simulink model "mpm_blocks"  (R2023a)
settings: Solver=VariableStepAuto  StartTime=0.0  StopTime=10.0  RelTol=1e-3
undefined symbols (not defined in the file or in its folder): conv, es
(part 3 of 3)

== system mpm_blocks/MOSFET w// Integrated Diode 2-Level VSC/Thermal Model/Subsystem4 ==
  P : Inport
  THS : Inport  Port=2
  Gain : Gain  Gain=1/(conv.dev(1).theta(4)+conv.theta(1))
  Gain1 : Gain  Gain=1/conv.dev(1).theta(3)
  Gain11 : Gain  Gain=1/conv.dev(1).c(1)
  Gain2 : Gain  Gain=1/conv.dev(1).c(4)
  Gain3 : Gain  Gain=1/conv.dev(1).theta(3)
  Gain4 : Gain  Gain=1/conv.dev(1).theta(2)
  Gain5 : Gain  Gain=1/conv.dev(1).c(3)
  Gain6 : Gain  Gain=1/conv.dev(1).theta(2)
  Gain7 : Gain  Gain=1/conv.dev(1).theta(1)
  Gain8 : Gain  Gain=1/conv.dev(1).c(2)
  Gain9 : Gain  Gain=1/conv.dev(1).theta(1)
  Integrator{,1..3} (4 alike) : Integrator  InitialCondition=conv.T_init-273.15
  Subtract{,1..9,11} (11 alike) : Sum  Inputs=+-
  T_c : Outport
  T_j : Outport  Port=2
  wires:
  [T2] -> Subtract4/1, Subtract6/1, Subtract7/2, Subtract9/2  "T2"
  Gain/1 -> Subtract2/2
  Subtract5/1 -> Gain5/1
  Gain4/1 -> Subtract5/1
  Subtract3/1 -> Gain3/1
  Gain8/1 -> Integrator1/1  "d_T2"
  Integrator/1 -> T_j/1, [T1]  "T1"
  [T3] -> Subtract1/1, Subtract3/1, Subtract4/2, Subtract6/2  "T3"
  P/1 -> Subtract11/1
  Subtract9/1 -> Gain9/1
  Subtract1/1 -> Gain1/1
  [T1] -> Subtract9/1, Subtract7/1  "T1"
  Integrator1/1 -> [T2]  "T2"
  Subtract/1 -> Gain/1
  [T4] -> Subtract/1, Subtract1/2, Subtract3/2  "T4"
  Subtract7/1 -> Gain7/1
  Subtract4/1 -> Gain4/1
  Integrator3/1 -> [T4], T_c/1  "T4"
  Gain2/1 -> Integrator3/1  "d_T4"
  Subtract8/1 -> Gain8/1
  THS/1 -> Subtract/2
  Gain1/1 -> Subtract2/1
  Gain9/1 -> Subtract11/2
  Gain3/1 -> Subtract5/2
  Integrator2/1 -> [T3]  "T3"
  Gain5/1 -> Integrator2/1  "d_T3"
  Gain11/1 -> Integrator/1  "d_T1"
  Subtract2/1 -> Gain2/1
  Subtract6/1 -> Gain6/1
  Subtract11/1 -> Gain11/1
  Gain7/1 -> Subtract8/1
  Gain6/1 -> Subtract8/2

== system mpm_blocks/MOSFET w// Integrated Diode 2-Level VSC/Thermal Model/Subsystem5 ==
  P : Inport
  THS : Inport  Port=2
  Gain : Gain  Gain=1/(conv.dev(1).theta(4)+conv.theta(1))
  Gain1 : Gain  Gain=1/conv.dev(1).theta(3)
  Gain11 : Gain  Gain=1/conv.dev(1).c(1)
  Gain2 : Gain  Gain=1/conv.dev(1).c(4)
  Gain3 : Gain  Gain=1/conv.dev(1).theta(3)
  Gain4 : Gain  Gain=1/conv.dev(1).theta(2)
  Gain5 : Gain  Gain=1/conv.dev(1).c(3)
  Gain6 : Gain  Gain=1/conv.dev(1).theta(2)
  Gain7 : Gain  Gain=1/conv.dev(1).theta(1)
  Gain8 : Gain  Gain=1/conv.dev(1).c(2)
  Gain9 : Gain  Gain=1/conv.dev(1).theta(1)
  Integrator{,1..3} (4 alike) : Integrator  InitialCondition=conv.T_init-273.15
  Subtract{,1..9,11} (11 alike) : Sum  Inputs=+-
  T_c : Outport
  T_j : Outport  Port=2
  wires:
  [T2] -> Subtract4/1, Subtract6/1, Subtract7/2, Subtract9/2  "T2"
  Gain/1 -> Subtract2/2
  Subtract5/1 -> Gain5/1
  Gain4/1 -> Subtract5/1
  Subtract3/1 -> Gain3/1
  Gain8/1 -> Integrator1/1  "d_T2"
  Integrator/1 -> T_j/1, [T1]  "T1"
  [T3] -> Subtract1/1, Subtract3/1, Subtract4/2, Subtract6/2  "T3"
  P/1 -> Subtract11/1
  Subtract9/1 -> Gain9/1
  Subtract1/1 -> Gain1/1
  [T1] -> Subtract9/1, Subtract7/1  "T1"
  Integrator1/1 -> [T2]  "T2"
  Subtract/1 -> Gain/1
  [T4] -> Subtract/1, Subtract1/2, Subtract3/2  "T4"
  Subtract7/1 -> Gain7/1
  Subtract4/1 -> Gain4/1
  Integrator3/1 -> [T4], T_c/1  "T4"
  Gain2/1 -> Integrator3/1  "d_T4"
  Subtract8/1 -> Gain8/1
  THS/1 -> Subtract/2
  Gain1/1 -> Subtract2/1
  Gain9/1 -> Subtract11/2
  Gain3/1 -> Subtract5/2
  Integrator2/1 -> [T3]  "T3"
  Gain5/1 -> Integrator2/1  "d_T3"
  Gain11/1 -> Integrator/1  "d_T1"
  Subtract2/1 -> Gain2/1
  Subtract6/1 -> Gain6/1
  Subtract11/1 -> Gain11/1
  Gain7/1 -> Subtract8/1
  Gain6/1 -> Subtract8/2

== system mpm_blocks/MOSFET w// Integrated Diode 2-Level VSC/Thermal Model/Subsystem6 ==
  P : Inport
  THS : Inport  Port=2
  Gain : Gain  Gain=1/(conv.dev(1).theta(4)+conv.theta(1))
  Gain1 : Gain  Gain=1/conv.dev(1).theta(3)
  Gain11 : Gain  Gain=1/conv.dev(1).c(1)
  Gain2 : Gain  Gain=1/conv.dev(1).c(4)
  Gain3 : Gain  Gain=1/conv.dev(1).theta(3)
  Gain4 : Gain  Gain=1/conv.dev(1).theta(2)
  Gain5 : Gain  Gain=1/conv.dev(1).c(3)
  Gain6 : Gain  Gain=1/conv.dev(1).theta(2)
  Gain7 : Gain  Gain=1/conv.dev(1).theta(1)
  Gain8 : Gain  Gain=1/conv.dev(1).c(2)
  Gain9 : Gain  Gain=1/conv.dev(1).theta(1)
  Integrator{,1..3} (4 alike) : Integrator  InitialCondition=conv.T_init-273.15
  Subtract{,1..9,11} (11 alike) : Sum  Inputs=+-
  T_c : Outport
  T_j : Outport  Port=2
  wires:
  [T2] -> Subtract4/1, Subtract6/1, Subtract7/2, Subtract9/2  "T2"
  Gain/1 -> Subtract2/2
  Subtract5/1 -> Gain5/1
  Gain4/1 -> Subtract5/1
  Subtract3/1 -> Gain3/1
  Gain8/1 -> Integrator1/1  "d_T2"
  Integrator/1 -> T_j/1, [T1]  "T1"
  [T3] -> Subtract1/1, Subtract3/1, Subtract4/2, Subtract6/2  "T3"
  P/1 -> Subtract11/1
  Subtract9/1 -> Gain9/1
  Subtract1/1 -> Gain1/1
  [T1] -> Subtract9/1, Subtract7/1  "T1"
  Integrator1/1 -> [T2]  "T2"
  Subtract/1 -> Gain/1
  [T4] -> Subtract/1, Subtract1/2, Subtract3/2  "T4"
  Subtract7/1 -> Gain7/1
  Subtract4/1 -> Gain4/1
  Integrator3/1 -> [T4], T_c/1  "T4"
  Gain2/1 -> Integrator3/1  "d_T4"
  Subtract8/1 -> Gain8/1
  THS/1 -> Subtract/2
  Gain1/1 -> Subtract2/1
  Gain9/1 -> Subtract11/2
  Gain3/1 -> Subtract5/2
  Integrator2/1 -> [T3]  "T3"
  Gain5/1 -> Integrator2/1  "d_T3"
  Gain11/1 -> Integrator/1  "d_T1"
  Subtract2/1 -> Gain2/1
  Subtract6/1 -> Gain6/1
  Subtract11/1 -> Gain11/1
  Gain7/1 -> Subtract8/1
  Gain6/1 -> Subtract8/2

== matlab function mpm_blocks/MOSFET w// Integrated Diode 2-Level VSC/Calculate Duty & Currents/Duty Cycle Estimation/MATLAB Function3 ==
  data: u input; y output
function y = checkMa(u)

if u > 1
    error('Modulation index (ma) greater than 1.');
end

y = u;

== matlab function mpm_blocks/MOSFET w// External Diode 2-Level VSC/Calculate Duty & Currents/Calculate Device Currents ==
  data: d_M input; d_deadTime input; i_s input; r_ds input; v_th input; r_dio input; i_M output size=[6 1]; i_D output size=[6 1]; d_D output
function [i_M, i_D, d_D]  = calcDevCurrent(d_M, d_deadTime, i_s, r_ds, v_th, r_dio)
%% Housekeeping
i_M = zeros(6,1);
i_D = zeros(6,1); 
d_D = zeros(6,1);
est_error = zeros(6,1);

v_ds_H = i_s .* r_ds(1:3); 
v_ds_L = -i_s .* r_ds(4:6); 

v_ds = [v_ds_H; v_ds_L];

%% A-Phase Devices 
% Devices (1) and (4)
% High-side
if(-v_ds(1) < v_th(1))
    i_M(1) = i_s(1); 
    i_D(1) = 0; 
    d_D(1) = d_deadTime;
else
    i_D(1) = -(i_s(1)*r_ds(1) + v_th(1)) / (r_ds(1) + r_dio(1));
    i_M(1) = i_s(1) + i_D(1); 
    d_D(1) = d_deadTime + d_M(1);
end

% Low-side
if(-v_ds(4) < v_th(4))
    i_M(4) = -i_s(1); 
    i_D(4) = 0; 
    d_D(4) = d_deadTime;
else
    i_D(4) = -(-i_s(1)*r_ds(4) + v_th(4)) / (r_ds(4) + r_dio(4));
    i_M(4) = i_D(4) - i_s(1); 
    d_D(4) = d_deadTime + d_M(4);
end

%% B-Phase Devices
% Devices (2) and (5)
% High-side
if(-v_ds(2) < v_th(2))
    i_M(2) = i_s(2); 
    i_D(2) = 0; 
    d_D(2) = d_deadTime;
else
    i_D(2) = -(i_s(2)*r_ds(2) + v_th(2)) / (r_ds(2) + r_dio(2));
    i_M(2) = i_s(2) + i_D(2); 
    d_D(2) = d_deadTime + d_M(2); 
end

% Low-side
if(-v_ds(5) < v_th(5))
    i_M(5) = -i_s(2); 
    i_D(5) = 0; 
    d_D(5) = d_deadTime; 
else
    i_D(5) = -(-i_s(2)*r_ds(5) + v_th(5)) / (r_ds(5) + r_dio(5));
    i_M(5) = i_D(5) - i_s(2); 
    d_D(5) = d_deadTime + d_M(5);
end

%% C-Phase Devices
% Devices (3) and (6)
% High-side
if(-v_ds(3) < v_th(3))
    i_M(3) = i_s(3); 
    i_D(3) = 0; 
    d_D(3) = d_deadTime; 
else
    i_D(3) = -(i_s(3)*r_ds(3) + v_th(3)) / (r_ds(3) + r_dio(3));
    i_M(3) = i_s(3) + i_D(3); 
    d_D(3) = d_deadTime + d_M(3); 
end

% Low-side
if(-v_ds(6) < v_th(3))
    i_M(6) = -i_s(3); 
    i_D(6) = 0; 
    d_D(6) = d_deadTime; 
else
    i_D(6) = -(-i_s(3)*r_ds(6) + v_th(6)) / (r_ds(6) + r_dio(6));
    i_M(6) = i_D(6) - i_s(3); 
    d_D(6) = d_deadTime + d_M(6); 
end

%% Calculate Error
for i = 1:3
    est_error(i) = i_s(i) - (i_M(i) - i_D(i));
    est_error(i+3) = i_s(i) + (i_M(i+3) - i_D(i+3));

    if(abs(est_error(i)/i_s(i)) > 0.2)
        error("CURRENT ESTIMATION ERROR: Estimation error for Device %d is greater than 20 percent", i)
    elseif(abs(est_error(i+3)/i_s(i)) > 0.2)
        error("CURRENT ESTIMATION ERROR: Estimation error for Device %d is greater than 20 percent", i)
    end
end

end

== matlab function mpm_blocks/IGBT 2-Level VSC2/Duty & Current Calculation/Calculate Device Currents ==
  data: d_Q input; d_deadTime input; i_s input; i_Q output size=[6 1]; d_Qnew output; i_D output size=[6 1]; d_D output
function [i_Q, d_Qnew, i_D, d_D]  = calcDevCurrent(d_Q, d_deadTime, i_s)
%% Housekeeping
i_Q = zeros(6,1);
i_D = zeros(6,1); 
d_D = zeros(6,1);
d_Qnew = zeros(6,1); 

% Calculating Device Currents
for i = 1:3
    if(i_s(i) > 0)
        % High-side device currents
        i_Q(i) = i_s(i); 
        i_D(i) = 0; 

        % Low-side device currents
        i_Q(i+3) = 0; 
        i_D(i+3) = i_s(i);

        % Diode duty cycle estimate
        d_Qnew(i) = d_Q(i);
        d_D(i) = 0;
        d_Qnew(i+3) = 0; 
        d_D(i+3) = d_Q(i+3) + d_deadTime;
    else
        % High-side device currents
        i_Q(i) = 0; 
        i_D(i) = -i_s(i); 

        % Low-side device currents
        i_Q(i+3) = -i_s(i); 
        i_D(i+3) = 0;

        % Diode duty cycle estimate
        d_Qnew(i) = 0; 
        d_D(i) = d_Q(i) + d_deadTime;
        d_Qnew(i+3) = d_Q(i+3);
        d_D(i+3) = 0; 
    end
end

== matlab function mpm_blocks/IGBT 2-Level VSC2/Duty & Current Calculation/MATLAB Function3 ==
  data: u input; y output
function y = checkMa(u)

if u > 1
    error('Modulation index (ma) greater than 1.');
end

y = u;

== matlab function mpm_blocks/MOSFET w// External Diode 2-Level VSC/Calculate Duty & Currents/Duty Cycle Estimation/MATLAB Function ==
  data: d1 input; d2 input; d3 input
function dutyCheck(d1, d2, d3)

if (d1+d2+d3 ~= 1)
    error("DUTY RATIO ERROR: check duty cycle function block")
end

== matlab function mpm_blocks/MOSFET w// External Diode 2-Level VSC/Calculate Duty & Currents/Duty Cycle Estimation/MATLAB Function3 ==
  data: u input; y output
function y = checkMa(u)

if u > 1
    error('Modulation index (ma) greater than 1.');
end

y = u;

== matlab function mpm_blocks/MOSFET w// Integrated Diode 2-Level VSC/Calculate Duty & Currents/Calculate Device Currents ==
  data: d_m input; d_d input; i_s input; r_ds input; v_th input; r_dio input; i_m output size=[6 1]; i_d output size=[6 1]; d_d_new output
function [i_m, i_d, d_d_new]  = calcDevCurrent(d_m, d_d, i_s, r_ds, v_th, r_dio)
%% Housekeeping
i_m = zeros(6,1);
i_d = zeros(6,1); 
d_d_new = zeros(6,1);
est_error = zeros(6,1);

v_ds_H = i_s .* r_ds(1:3); 
v_ds_L = -i_s .* r_ds(4:6); 

v_ds = [v_ds_H; v_ds_L];

%% A-Phase Devices 
% Devices (1) and (4)
% High-side
if(-v_ds(1) < v_th(1))
    i_m(1) = i_s(1); 
    i_d(1) = 0; 
    d_d_new(1) = d_d;
else
    i_d(1) = -(i_s(1)*r_ds(1) + v_th(1)) / (r_ds(1) + r_dio(1));
    i_m(1) = i_s(1) + i_d(1); 
    d_d_new(1) = d_d + d_m(1);
end

% Low-side
if(-v_ds(4) < v_th(4))
    i_m(4) = -i_s(1); 
    i_d(4) = 0; 
    d_d_new(4) = d_d;
else
    i_d(4) = -(-i_s(1)*r_ds(4) + v_th(4)) / (r_ds(4) + r_dio(4));
    i_m(4) = i_d(4) - i_s(1); 
    d_d_new(4) = d_d + d_m(4);
end

%% B-Phase Devices
% Devices (2) and (5)
% High-side
if(-v_ds(2) < v_th(2))
    i_m(2) = i_s(2); 
    i_d(2) = 0; 
    d_d_new(2) = d_d;
else
    i_d(2) = -(i_s(2)*r_ds(2) + v_th(2)) / (r_ds(2) + r_dio(2));
    i_m(2) = i_s(2) + i_d(2); 
    d_d_new(2) = d_d + d_m(2); 
end

% Low-side
if(-v_ds(5) < v_th(5))
    i_m(5) = -i_s(2); 
    i_d(5) = 0; 
    d_d_new(5) = d_d; 
else
    i_d(5) = -(-i_s(2)*r_ds(5) + v_th(5)) / (r_ds(5) + r_dio(5));
    i_m(5) = i_d(5) - i_s(2); 
    d_d_new(5) = d_d + d_m(5);
end

%% C-Phase Devices
% Devices (3) and (6)
% High-side
if(-v_ds(3) < v_th(3))
    i_m(3) = i_s(3); 
    i_d(3) = 0; 
    d_d_new(3) = d_d; 
else
    i_d(3) = -(i_s(3)*r_ds(3) + v_th(3)) / (r_ds(3) + r_dio(3));
    i_m(3) = i_s(3) + i_d(3); 
    d_d_new(3) = d_d + d_m(3); 
end

% Low-side
if(-v_ds(6) < v_th(3))
    i_m(6) = -i_s(3); 
    i_d(6) = 0; 
    d_d_new(6) = d_d; 
else
    i_d(6) = -(-i_s(3)*r_ds(6) + v_th(6)) / (r_ds(6) + r_dio(6));
    i_m(6) = i_d(6) - i_s(3); 
    d_d_new(6) = d_d + d_m(6); 
end

%% Calculate Error
for i = 1:3
    est_error(i) = i_s(i) - (i_m(i) - i_d(i));
    est_error(i+3) = i_s(i) + (i_m(i+3) - i_d(i+3));

    if(abs(est_error(i)/i_s(i)) > 0.2)
        error("CURRENT ESTIMATION ERROR: Estimation error for Device %d is greater than 20 percent", i)
    elseif(abs(est_error(i+3)/i_s(i)) > 0.2)
        error("CURRENT ESTIMATION ERROR: Estimation error for Device %d is greater than 20 percent", i)
    end
end

end

== matlab function mpm_blocks/MOSFET w// Integrated Diode 2-Level VSC/Calculate Duty & Currents/Duty Cycle Estimation/MATLAB Function ==
  data: d1 input; d2 input; d3 input
function dutyCheck(d1, d2, d3)

if (d1+d2+d3 ~= 1)
    error("DUTY RATIO ERROR: check duty cycle function block")
end
